simulink model "Completo"  (R2022a)
settings: Solver=VariableStepAuto  StartTime=0.0  StopTime=8  RelTol=1e-3
values from neighbouring files (symbols this model uses):
  A = sys.A    [RealEstadoObserServoTipo0.m]
  B = sys.B    [RealEstadoObserServoTipo0.m]
  C = sys.C    [RealEstadoObserServoTipo0.m]    (also in control 2 tf.mat = 0.0033)
  Ke = acker(A',C',[-30 -30 -30])'    [RealEstadoObserServoTipo0.m]
  Khat = acker(Ahat,Bhat,J)    [RealEstadoObserServoTipo0.m]
settings Model: Creator=Juan Andres  LastModifiedBy=paoli
settings SolverCC: AlgebraicLoopSolver=TrustRegion
settings DebuggingCC: UnconnectedInputMsg=warning  UnconnectedOutputMsg=warning  UnconnectedLineMsg=warning  SFMachineParentedDataDiag=warning

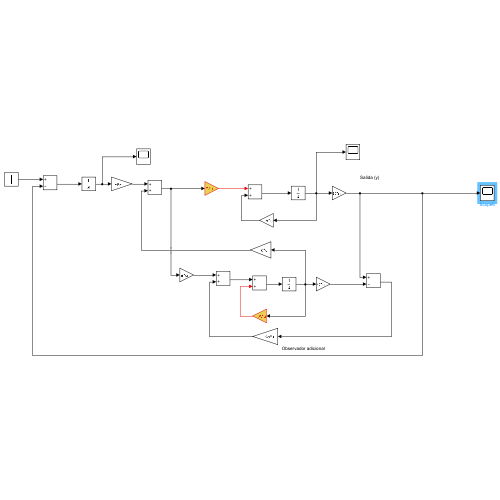
[thumbnail: Simulink's stored preview of the top-level diagram]
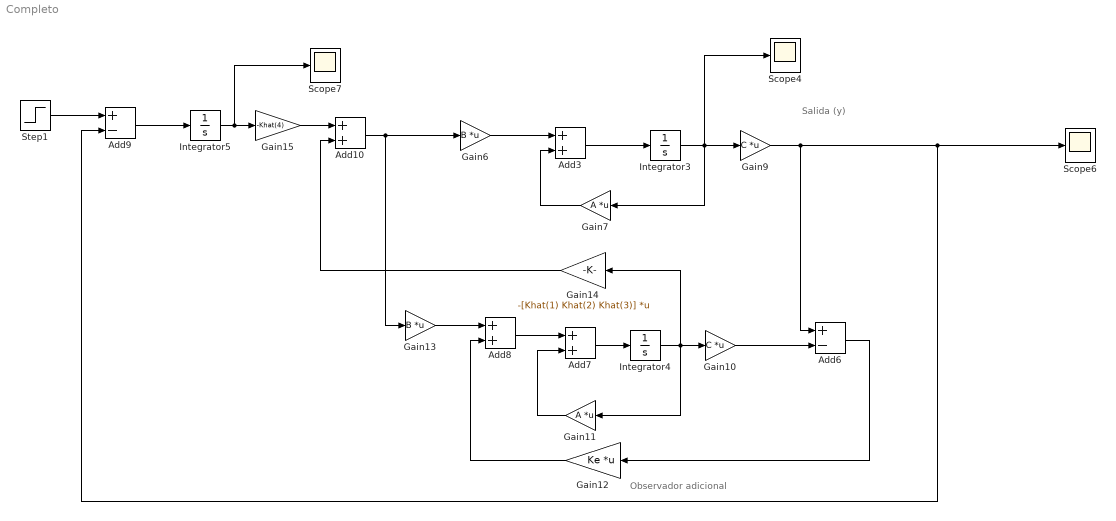
== system Completo ==
  note: Salida (y)
  note: Observador adicional
  Add{3,7..8,10} (4 alike) : Sum
  Add6 : Sum  Inputs=+-
  Add9 : Sum  Inputs=+-
  Gain10 : Gain  Gain=C  Multiplication=Matrix(K*u)
  Gain11 : Gain  Gain=A  Multiplication=Matrix(K*u)
  Gain12 : Gain  Gain=Ke  Multiplication=Matrix(K*u)
  Gain13 : Gain  Gain=B  Multiplication=Matrix(K*u)
  Gain14 : Gain  Gain=-[Khat(1) Khat(2) Khat(3)]  Multiplication=Matrix(K*u)
  Gain15 : Gain  Gain=-Khat(4)
  Gain6 : Gain  Gain=B  Multiplication=Matrix(K*u)
  Gain7 : Gain  Gain=A  Multiplication=Matrix(K*u)
  Gain9 : Gain  Gain=C  Multiplication=Matrix(K*u)
  Integrator3 : Integrator  InitialCondition=[0;0;0]
  Integrator4 : Integrator  InitialCondition=[0;0;0]
  Integrator5 : Integrator
  Scope4 : Scope
  Scope6 : Scope
  Scope7 : Scope
  Step1 : Step  Time=0  SampleTime=0
  wires:
  Gain14/1 -> Add10/2
  Gain10/1 -> Add6/2
  Add6/1 -> Gain12/1
  Add3/1 -> Integrator3/1
  Integrator4/1 -> Gain11/1, Gain14/1, Gain10/1
  Add8/1 -> Add7/1
  Gain13/1 -> Add8/1
  Gain11/1 -> Add7/2
  Integrator3/1 -> Scope4/1, Gain9/1, Gain7/1
  Add7/1 -> Integrator4/1
  Gain6/1 -> Add3/1
  Gain12/1 -> Add8/2
  Gain7/1 -> Add3/2
  Integrator5/1 -> Scope7/1, Gain15/1
  Step1/1 -> Add9/1
  Gain9/1 -> Add6/1, Add9/2, Scope6/1
  Add9/1 -> Integrator5/1
  Gain15/1 -> Add10/1
  Add10/1 -> Gain6/1, Gain13/1
